simulink model "fxpdemo_sfun_user_asr"  (Simulink 5.0)
settings: Solver=FixedStepDiscrete  StartTime=0.0  StopTime=1  FixedStep=0.001  RelTol=1e-3
libraries: fixpt_lib_4 x7
settings Model: Creator=andyb  LastModifiedBy=andyb  ExtModeAutoUpdateStatusClock=off  ParameterPrecisionLossMsg=none  RTWInlineParameters=on  RTWOptions="-aEnforceIntegerDowncast=1 -aExtMode=0 -aExtModeTesting=0 -aFoldNonRolledExpr=1 -aForceParamTrailComments=0 -aGenerateComments=1 -aGenerateFullHeader=1 -aGenerateReport=1 -aIgnoreCustomStorageClasses=1 -aIncDataTypeInIds=0 -aIncHierarchyInIds=0 -aInlineInvariantSignals=0 -aInlineParameters=1 -aInlinedPrmAccess=\"Literals\" -aLocalBlockOutputs=1 -aLogVarNameModifier=\"rt_\" -aMaxRTWIdLen=31 -aPrefixModelToSubsysFcnNames=1 -aRTWVerbose=1 -aRollThreshold=5 -aShowEliminatedStatements=0"

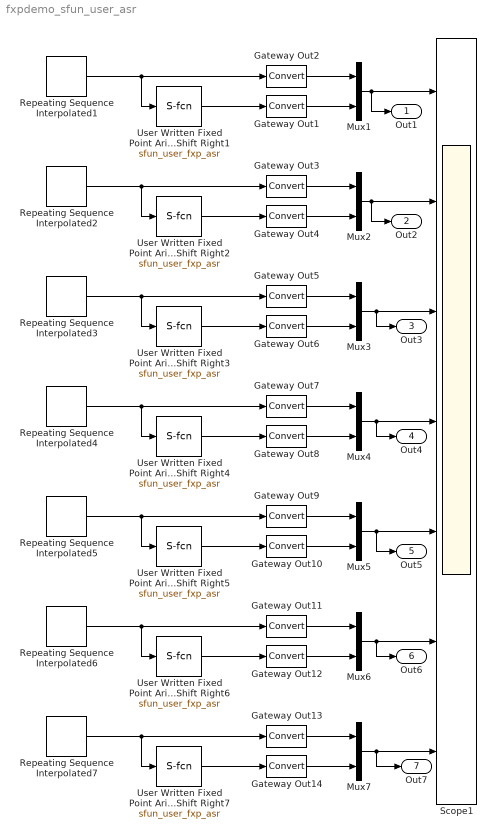
== system fxpdemo_sfun_user_asr ==
  Gateway Out{1..14} (14 alike) : DataTypeConversion  DataType=double
  Mux{1..7} (7 alike) : Mux  Inputs=2
  Repeating Sequence Interpolated1 : fixpt_lib_4/Sources/Repeating Sequence Interpolated  OutValues=0+2*[0 0.25 0.5 0.75 1].'  TimeValues=[0 0.25 0.5 0.75 1].'  LookUpMeth=Interpolation-Use End Values  tsamp=0.001  OutputDataTypeScalingMode=Specify via dialog  OutDataType=ufix(8)  OutScaling=2^-7
  Repeating Sequence Interpolated2 : fixpt_lib_4/Sources/Repeating Sequence Interpolated  OutValues=-2+4*[0 0.25 0.5 0.75 1].'  TimeValues=[0 0.25 0.5 0.75 1].'  LookUpMeth=Interpolation-Use End Values  tsamp=0.001  OutputDataTypeScalingMode=Specify via dialog  OutDataType=sfix(8)  OutScaling=2^-6
  Repeating Sequence Interpolated3 : fixpt_lib_4/Sources/Repeating Sequence Interpolated  OutValues=0+2*[0 0.25 0.5 0.75 1].'  TimeValues=[0 0.25 0.5 0.75 1].'  LookUpMeth=Interpolation-Use End Values  tsamp=0.001  OutputDataTypeScalingMode=Specify via dialog  OutDataType=ufix(16)  OutScaling=2^-15
  Repeating Sequence Interpolated4 : fixpt_lib_4/Sources/Repeating Sequence Interpolated  OutValues=-2+4*[0 0.25 0.5 0.75 1].'  TimeValues=[0 0.25 0.5 0.75 1].'  LookUpMeth=Interpolation-Use End Values  tsamp=0.001  OutputDataTypeScalingMode=Specify via dialog  OutDataType=sfix(16)  OutScaling=2^-14
  Repeating Sequence Interpolated5 : fixpt_lib_4/Sources/Repeating Sequence Interpolated  OutValues=0+2*[0 0.25 0.5 0.75 1].'  TimeValues=[0 0.25 0.5 0.75 1].'  LookUpMeth=Interpolation-Use End Values  tsamp=0.001  OutputDataTypeScalingMode=Specify via dialog  OutDataType=ufix(32)  OutScaling=2^-31
  Repeating Sequence Interpolated6 : fixpt_lib_4/Sources/Repeating Sequence Interpolated  OutValues=-2+4*[0 0.25 0.5 0.75 1].'  TimeValues=[0 0.25 0.5 0.75 1].'  LookUpMeth=Interpolation-Use End Values  tsamp=0.001  OutputDataTypeScalingMode=Specify via dialog  OutDataType=sfix(32)  OutScaling=2^-30
  Repeating Sequence Interpolated7 : fixpt_lib_4/Sources/Repeating Sequence Interpolated  OutValues=-2+4*[0 0.25 0.5 0.75 1].'  TimeValues=[0 0.25 0.5 0.75 1].'  LookUpMeth=Interpolation-Use End Values  tsamp=0.001  OutputDataTypeScalingMode=Specify via dialog  OutDataType=sfix(12)  OutScaling=2^-10
  Scope1 : Scope  NumInputPorts=7
      settings: TimeRange=1  YMin=0~-2~0~-2~0~-2~-2  YMax=2~2~2~2~2~2~2
  User Written Fixed Point Arithmetic Shift Right1 : S-Function  FunctionName=sfun_user_fxp_asr  Parameters=numBitsShiftRight  mask(User ASR){numBitsShiftRight=6}
      mask prompts: numBitsShiftRight "Number of Bits to Shift Right Bits and Binary Point"
      mask help: Arithmetic Shift Right
      mask Display: disp(sprintf('ASR %d',numBitsShiftRight))
  User Written Fixed Point Arithmetic Shift Right2 : S-Function  FunctionName=sfun_user_fxp_asr  Parameters=numBitsShiftRight  mask(User ASR){numBitsShiftRight=5}
      mask prompts: numBitsShiftRight "Number of Bits to Shift Right Bits and Binary Point"
      mask help: Arithmetic Shift Right
      mask Display: disp(sprintf('ASR %d',numBitsShiftRight))
  User Written Fixed Point Arithmetic Shift Right3 : S-Function  FunctionName=sfun_user_fxp_asr  Parameters=numBitsShiftRight  mask(User ASR){numBitsShiftRight=14}
      mask prompts: numBitsShiftRight "Number of Bits to Shift Right Bits and Binary Point"
      mask help: Arithmetic Shift Right
      mask Display: disp(sprintf('ASR %d',numBitsShiftRight))
  User Written Fixed Point Arithmetic Shift Right4 : S-Function  FunctionName=sfun_user_fxp_asr  Parameters=numBitsShiftRight  mask(User ASR){numBitsShiftRight=13}
      mask prompts: numBitsShiftRight "Number of Bits to Shift Right Bits and Binary Point"
      mask help: Arithmetic Shift Right
      mask Display: disp(sprintf('ASR %d',numBitsShiftRight))
  User Written Fixed Point Arithmetic Shift Right5 : S-Function  FunctionName=sfun_user_fxp_asr  Parameters=numBitsShiftRight  mask(User ASR){numBitsShiftRight=30}
      mask prompts: numBitsShiftRight "Number of Bits to Shift Right Bits and Binary Point"
      mask help: Arithmetic Shift Right
      mask Display: disp(sprintf('ASR %d',numBitsShiftRight))
  User Written Fixed Point Arithmetic Shift Right6 : S-Function  FunctionName=sfun_user_fxp_asr  Parameters=numBitsShiftRight  mask(User ASR){numBitsShiftRight=29}
      mask prompts: numBitsShiftRight "Number of Bits to Shift Right Bits and Binary Point"
      mask help: Arithmetic Shift Right
      mask Display: disp(sprintf('ASR %d',numBitsShiftRight))
  User Written Fixed Point Arithmetic Shift Right7 : S-Function  FunctionName=sfun_user_fxp_asr  Parameters=numBitsShiftRight  mask(User ASR){numBitsShiftRight=8}
      mask prompts: numBitsShiftRight "Number of Bits to Shift Right Bits and Binary Point"
      mask help: Arithmetic Shift Right
      mask Display: disp(sprintf('ASR %d',numBitsShiftRight))
  Out1 : Outport
  Out2 : Outport  Port=2
  Out3 : Outport  Port=3
  Out4 : Outport  Port=4
  Out5 : Outport  Port=5
  Out6 : Outport  Port=6
  Out7 : Outport  Port=7
  wires:
  Repeating Sequence Interpolated1/1 -> Gateway Out2/1, User Written Fixed Point Arithmetic Shift Right1/1
  User Written Fixed Point Arithmetic Shift Right1/1 -> Gateway Out1/1
  Mux1/1 -> Scope1/1, Out1/1
  Gateway Out2/1 -> Mux1/1
  Gateway Out1/1 -> Mux1/2
  Repeating Sequence Interpolated2/1 -> User Written Fixed Point Arithmetic Shift Right2/1, Gateway Out3/1
  User Written Fixed Point Arithmetic Shift Right2/1 -> Gateway Out4/1
  Gateway Out3/1 -> Mux2/1
  Gateway Out4/1 -> Mux2/2
  Mux2/1 -> Scope1/2, Out2/1
  Repeating Sequence Interpolated3/1 -> User Written Fixed Point Arithmetic Shift Right3/1, Gateway Out5/1
  User Written Fixed Point Arithmetic Shift Right3/1 -> Gateway Out6/1
  Gateway Out5/1 -> Mux3/1
  Gateway Out6/1 -> Mux3/2
  Repeating Sequence Interpolated4/1 -> User Written Fixed Point Arithmetic Shift Right4/1, Gateway Out7/1
  User Written Fixed Point Arithmetic Shift Right4/1 -> Gateway Out8/1
  Gateway Out7/1 -> Mux4/1
  Gateway Out8/1 -> Mux4/2
  Repeating Sequence Interpolated5/1 -> User Written Fixed Point Arithmetic Shift Right5/1, Gateway Out9/1
  User Written Fixed Point Arithmetic Shift Right5/1 -> Gateway Out10/1
  Gateway Out9/1 -> Mux5/1
  Gateway Out10/1 -> Mux5/2
  Repeating Sequence Interpolated6/1 -> User Written Fixed Point Arithmetic Shift Right6/1, Gateway Out11/1
  User Written Fixed Point Arithmetic Shift Right6/1 -> Gateway Out12/1
  Gateway Out11/1 -> Mux6/1
  Gateway Out12/1 -> Mux6/2
  Repeating Sequence Interpolated7/1 -> User Written Fixed Point Arithmetic Shift Right7/1, Gateway Out13/1
  User Written Fixed Point Arithmetic Shift Right7/1 -> Gateway Out14/1
  Gateway Out13/1 -> Mux7/1
  Gateway Out14/1 -> Mux7/2
  Mux3/1 -> Scope1/3, Out3/1
  Mux4/1 -> Scope1/4, Out4/1
  Mux5/1 -> Scope1/5, Out5/1
  Mux6/1 -> Scope1/6, Out6/1
  Mux7/1 -> Scope1/7, Out7/1
